simulink model "Simulacio_de_sistemas_Discretos"  (R2017a)
settings: Solver=VariableStepAuto  StartTime=0.0  StopTime=10.0  RelTol=1e-3
libraries: simulink x4
settings Model: Creator=franj  LastModifiedBy=franj

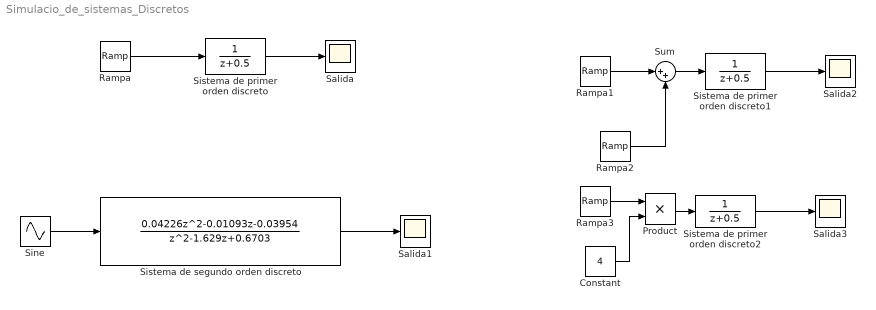
== system Simulacio_de_sistemas_Discretos ==
  Constant : Constant  Value=4
  Product : Product
  Rampa{,1..3} (4 alike) : simulink/Sources/Ramp  slope=1  start=0  X0=0
  Salida{,1..3} (4 alike) : Scope
  "Sine " : Sin  SampleTime=0
  Sistema de primer orden discreto : DiscreteTransferFcn
  Sistema de primer orden discreto1 : DiscreteTransferFcn
  Sistema de primer orden discreto2 : DiscreteTransferFcn
  Sistema de segundo orden discreto : DiscreteTransferFcn  Numerator=[0.04226 -0.01093 -0.03954]  Denominator=[1 -1.629 0.6703]
  Sum : Sum  Inputs=|++
  wires:
  Rampa/1 -> Sistema de primer orden discreto/1
  Sistema de primer orden discreto/1 -> Salida/1
  Sistema de segundo orden discreto/1 -> Salida1/1
  "Sine "/1 -> Sistema de segundo orden discreto/1
  Sistema de primer orden discreto1/1 -> Salida2/1
  Rampa1/1 -> Sum/1
  Sum/1 -> Sistema de primer orden discreto1/1
  Rampa2/1 -> Sum/2
  Sistema de primer orden discreto2/1 -> Salida3/1
  Product/1 -> Sistema de primer orden discreto2/1
  Rampa3/1 -> Product/1
  Constant/1 -> Product/2
